simulink model "inverter_w_BESS"  (R2024b)
settings: Solver=VariableStepAuto  StartTime=0.0  StopTime=4  RelTol=1e-3
undefined symbols (not defined in the file): Batt, BatteryCallback, DiscIntNeverNeededParam, gcbh, Q, sps_rtmsupport, Ts, Ts_Control
libraries: simulink x12, spsSeriesRLCBranchLib x7, slpidlib x6, ee_lib x5, nesl_utility x5, eePowerMeasurement x3, powerlib_extras x3, spsCurrentVoltageSimscapeInterfaceLib x3, spsThreePhaseVIMeasurementLib x2, spsCurrentMeasurementLib x2, spsGroundLib x2, spsThreePhaseSeriesRLCBranchLib x2
(part 2 of 2)

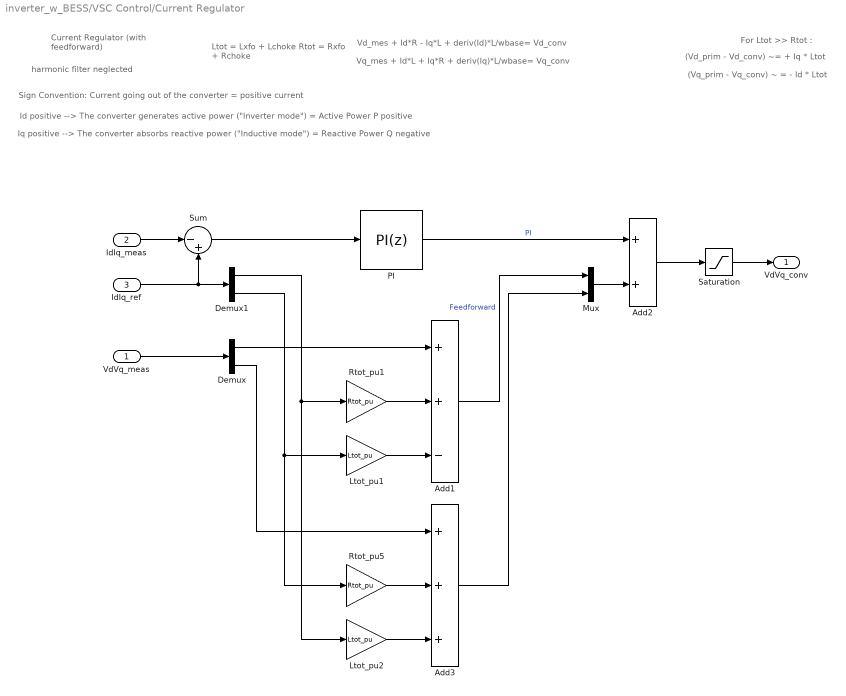
== system inverter_w_BESS/VSC Control/Current Regulator ==
  note: For Ltot >> Rtot :
  note: (Vq_prim - Vq_conv) ~ = - Id * Ltot
  note: (Vd_prim - Vd_conv) ~= + Iq * Ltot
  note: Ltot = Lxfo + Lchoke
      | Rtot = Rxfo + Rchoke
  note: Id positive --> The converter generates active power ("Inverter mode") = Active Power P positive
  note: Iq positive --> The converter absorbs reactive power ("Inductive mode") = Reactive Power Q negative
  note: Sign Convention: Current going out of the converter = positive current
  note: Current Regulator
      | (with feedforward)
  note: Vq_mes + Id*L + Iq*R + deriv(Iq)*L/wbase= Vq_conv
  note: Vd_mes + Id*R - Iq*L + deriv(Id)*L/wbase= Vd_conv
  note: harmonic filter neglected
  VdVq_meas : Inport  PortDimensions=2
  IdIq_meas : Inport  Port=2  PortDimensions=2
  IdIq_ref : Inport  Port=3  PortDimensions=2
  Add1 : Sum  Inputs=++-
  Add2 : Sum
  Add3 : Sum  Inputs=+++
  Demux : Demux  Outputs=2
  Demux1 : Demux  Outputs=2
  Ltot_pu1 : Gain  Gain=Ltot_pu  SaturateOnIntegerOverflow=on  OutDataTypeStr=Inherit: Same as input  ParamDataTypeStr=Inherit: Same as input
  Ltot_pu2 : Gain  Gain=Ltot_pu  SaturateOnIntegerOverflow=on  OutDataTypeStr=Inherit: Same as input  ParamDataTypeStr=Inherit: Same as input
  Mux : Mux  Inputs=2
  PI : slpidlib/PID Controller  Controller=PI  Form=Parallel  TimeDomain=Discrete-time  UseExternalTs=off  SampleTime=Ts  IntegratorMethod=Forward Euler  FilterMethod=Forward Euler  ControllerParametersSource=internal  P=Kp_Ireg  I=Ki_Ireg  UseKiTs=off  D=0  UseExternalDerivativeSource=off  N=100  UseFilter=on  TunerSelectOption=Transfer Function Based (PID Tuner App)  InitialConditionSource=internal  InitialConditionForIntegrator=0  InitialConditionForFilter=0  DifferentiatorICPrevScaledInput=0  ExternalReset=none  TrackingMode=off  Kt=1  LimitOutput=on  SatLimitsSource=internal  UpperSaturationLimit=2  LowerSaturationLimit=-2  LinearizeAsGain=off  AntiWindupMode=none  Kb=1  LimitIntegrator=off  UpperIntegratorSaturationLimit=inf  LowerIntegratorSaturationLimit=-inf  POutMin=[]  POutMax=[]  IOutMin=[]  IOutMax=[]  DOutMin=[]  DOutMax=[]  NOutMin=[]  NOutMax=[]  SumOutMin=[]  SumOutMax=[]  SaturationOutMin=[]  SaturationOutMax=[]  PParamMin=[]  PParamMax=[]  IParamMin=[]  IParamMax=[]  DParamMin=[]  DParamMax=[]  NParamMin=[]  NParamMax=[]  KbParamMin=[]  KbParamMax=[]  KtParamMin=[]  KtParamMax=[]  KbOutMin=[]  KbOutMax=[]  KtOutMin=[]  KtOutMax=[]  IntegratorOutMin=[]  IntegratorOutMax=[]  FilterOutMin=[]  FilterOutMax=[]  SumI1OutMin=[]  SumI1OutMax=[]  SumI2OutMin=[]  SumI2OutMax=[]  SumI3OutMin=[]  SumI3OutMax=[]  SumI4OutMin=[]  SumI4OutMax=[]  SumDOutMin=[]  SumDOutMax=[]  DifferentiatorOutMin=[]  DifferentiatorOutMax=[]  FilterDiffOutCoefMin=[]  FilterDiffOutCoefMax=[]  ReciprocalOutMin=[]  ReciprocalOutMax=[]  SumDenOutMin=[]  SumDenOutMax=[]  SumNumOutMin=[]  SumNumOutMax=[]  DivideOutMin=[]  DivideOutMax=[]  UdiffTsProdOutMin=[]  UdiffTsProdOutMax=[]  NTsProdOutMin=[]  NTsProdOutMax=[]  UintegralTsProdOutMin=[]  UintegralTsProdOutMax=[]  UngainTsProdOutMin=[]  UngainTsProdOutMax=[]  ClampingZeroOutDataTypeStr=Inherit: Inherit via back propagation  ClampingZeroOutMin=[]  ClampingZeroOutMax=[]  FilterDenConstantOutDataTypeStr=Inherit: Inherit via back propagation  FilterDenConstantOutMin=[]  FilterDenConstantOutMax=[]  PCopyOutDataTypeStr=Inherit: Inherit via back propagation  PCopyOutMin=[]  PCopyOutMax=[]  NCopyOutDataTypeStr=Inherit: Inherit via back propagation  NCopyOutMin=[]  NCopyOutMax=[]  IntegratorContinuousStateAttributes=''  IntegratorStateMustResolveToSignalObject=off  IntegratorRTWStateStorageClass=Auto  FilterContinuousStateAttributes=''  FilterStateMustResolveToSignalObject=off  FilterRTWStateStorageClass=Auto  ParallelPVariant=InternalParameters  IdealPVariant=Disabled  IVariant=InternalParameters  DVariant=Disabled  IntegratorVariant=Discrete  SatVariant=Enabled  AWVariant=Passthrough  PCopyVariant=Disabled  TRVariant=Disabled  FdbkBlocksVariant=Forward  IdealPFdbkVariant=Disabled  SatFdbkVariant=Disabled  DerivativeFilterVariant=Disabled  NVariant=Disabled  NCopyVariant=Disabled_SignalSpec  FilterICVariant=Disabled  IntegratorICVariant=InternalICs  ExternalResetVariant=Disabled  TRSumVariant=Passthrough  SumFdbkVariant=Disabled  SumVariant=Sum_PI  TsampFilterVariant=InternalTs  TsampNgainVariant=Passthrough  TsampIntegralVariant=Disabled_SignalSpec  ExternalSaturationOutDataTypeStr=Inherit: Same as second input  DerivativeSourceVariant=Disabled  PreIntVariant=InternalPreInt
  Rtot_pu1 : Gain  Gain=Rtot_pu  SaturateOnIntegerOverflow=on  OutDataTypeStr=Inherit: Same as input  ParamDataTypeStr=Inherit: Same as input
  Rtot_pu5 : Gain  Gain=Rtot_pu  SaturateOnIntegerOverflow=on  OutDataTypeStr=Inherit: Same as input  ParamDataTypeStr=Inherit: Same as input
  Saturation : Saturate  UpperLimit=2  LowerLimit=-2
  Sum : Sum  Inputs=|-+
  VdVq_conv : Outport  VectorParamsAs1DForOutWhenUnconnected=off
  wires:
  Add3/1 -> Mux/2
  Demux/2 -> Add3/1
  Add1/1 -> Mux/1  "Feedforward"
  Ltot_pu2/1 -> Add3/3
  Rtot_pu5/1 -> Add3/2
  Demux1/2 -> Rtot_pu5/1, Ltot_pu1/1
  Ltot_pu1/1 -> Add1/3
  Demux1/1 -> Ltot_pu2/1, Rtot_pu1/1
  Rtot_pu1/1 -> Add1/2
  Demux/1 -> Add1/1
  VdVq_meas/1 -> Demux/1
  Saturation/1 -> VdVq_conv/1
  Add2/1 -> Saturation/1
  IdIq_meas/1 -> Sum/1
  IdIq_ref/1 -> Demux1/1, Sum/2
  Sum/1 -> PI/1
  PI/1 -> Add2/1  "PI"
  Mux/1 -> Add2/2

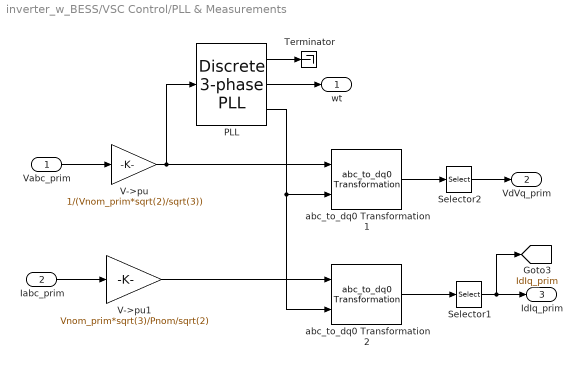
== system inverter_w_BESS/VSC Control/PLL & Measurements ==
  Vabc_prim : Inport
  Iabc_prim : Inport  Port=2
  PLL : powerlib_extras/Discrete  Control Blocks/Discrete 3-phase PLL  Fmin=45  Par_Init="[-0.57  Fnom]"  ParK=[60 1400]  Ts=Ts  AGC=off
  Selector1 : Selector  InputPortWidth=3  IndexOptions=Index vector (dialog)  Indices=[1 2]  OutputSizes=1
  Selector2 : Selector  InputPortWidth=3  IndexOptions=Index vector (dialog)  Indices=[1 2]  OutputSizes=1
  Terminator : Terminator
  V->pu : Gain  Gain=1/(Vnom_prim*sqrt(2)/sqrt(3))  SaturateOnIntegerOverflow=on  OutDataTypeStr=Inherit: Same as input  ParamDataTypeStr=Inherit: Same as input
  V->pu1 : Gain  Gain=Vnom_prim*sqrt(3)/Pnom/sqrt(2)  SaturateOnIntegerOverflow=on  OutDataTypeStr=Inherit: Same as input  ParamDataTypeStr=Inherit: Same as input
  abc_to_dq0 Transformation1 : powerlib_extras/Measurements/abc_to_dq0 Transformation
  abc_to_dq0 Transformation2 : powerlib_extras/Measurements/abc_to_dq0 Transformation
  wt : Outport  VectorParamsAs1DForOutWhenUnconnected=off
  VdVq_prim : Outport  Port=2  VectorParamsAs1DForOutWhenUnconnected=off
  IdIq_prim : Outport  Port=3  VectorParamsAs1DForOutWhenUnconnected=off
  tag scope: IdIq_prim=global
  wires:
  PLL/1 -> Terminator/1
  PLL/3 -> abc_to_dq0 Transformation1/2, abc_to_dq0 Transformation2/2
  Selector1/1 -> IdIq_prim/1, [IdIq_prim]
  Selector2/1 -> VdVq_prim/1
  abc_to_dq0 Transformation1/1 -> Selector2/1
  Iabc_prim/1 -> V->pu1/1
  Vabc_prim/1 -> V->pu/1
  PLL/2 -> wt/1
  abc_to_dq0 Transformation2/1 -> Selector1/1
  V->pu/1 -> abc_to_dq0 Transformation1/1, PLL/1
  V->pu1/1 -> abc_to_dq0 Transformation2/1

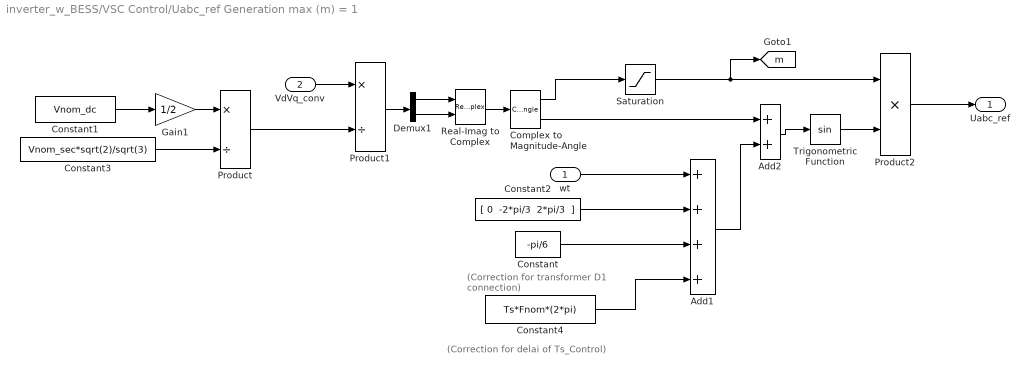
== system inverter_w_BESS/VSC Control/Uabc_ref Generation max (m) = 1 ==
  note: (Correction for delai of Ts_Control)
  note: (Correction for transformer
      |  D1 connection)
  wt : Inport
  VdVq_conv : Inport  Port=2
  Add1 : Sum  Inputs=++++
  Add2 : Sum
  Complex to Magnitude-Angle : ComplexToMagnitudeAngle
  Constant : Constant  Value=-pi/6
  Constant1 : Constant  Value=Vnom_dc
  Constant2 : Constant  Value="[ 0  -2*pi/3  2*pi/3  ]"
  Constant3 : Constant  Value=Vnom_sec*sqrt(2)/sqrt(3)
  Constant4 : Constant  Value=Ts*Fnom*(2*pi)
  Demux1 : Demux  Outputs=2
  Gain1 : Gain  Gain=1/2
  Product : Product  Inputs=*/  RndMeth=Zero
  Product1 : Product  Inputs=*/  RndMeth=Zero
  Product2 : Product  Inputs=**  RndMeth=Zero
  Real-Imag to Complex : RealImagToComplex
  Saturation : Saturate  UpperLimit=1  LowerLimit=0
  Trigonometric Function : Trigonometry
  Uabc_ref : Outport  VectorParamsAs1DForOutWhenUnconnected=off
  tag scope: m=global
  wires:
  Constant4/1 -> Add1/4
  wt/1 -> Add1/1
  Product2/1 -> Uabc_ref/1
  Trigonometric Function/1 -> Product2/2
  Saturation/1 -> Product2/1, [m]
  Add2/1 -> Trigonometric Function/1
  Add1/1 -> Add2/2
  Complex to Magnitude-Angle/2 -> Add2/1
  Product/1 -> Product1/2
  Constant3/1 -> Product/2
  Constant/1 -> Add1/3
  Constant2/1 -> Add1/2
  Demux1/2 -> Real-Imag to Complex/2
  Demux1/1 -> Real-Imag to Complex/1
  Real-Imag to Complex/1 -> Complex to Magnitude-Angle/1
  Gain1/1 -> Product/1
  Product1/1 -> Demux1/1
  VdVq_conv/1 -> Product1/1
  Constant1/1 -> Gain1/1
  Complex to Magnitude-Angle/1 -> Saturation/1

== system inverter_w_BESS/VSC Control/VDC Regulator ==
  Vdc_meas : Inport  PortDimensions=1
  Vdc_ref : Inport  Port=2  PortDimensions=1
  PI : slpidlib/PID Controller  Controller=PI  Form=Parallel  TimeDomain=Discrete-time  UseExternalTs=off  SampleTime=Ts  IntegratorMethod=Trapezoidal  FilterMethod=Forward Euler  ControllerParametersSource=internal  P=Kp_VDCreg  I=Ki_VDCreg  UseKiTs=off  D=0  UseExternalDerivativeSource=off  N=100  UseFilter=on  TunerSelectOption=Transfer Function Based (PID Tuner App)  InitialConditionSource=internal  InitialConditionForIntegrator=0  InitialConditionForFilter=0  DifferentiatorICPrevScaledInput=0  ExternalReset=none  TrackingMode=off  Kt=1  LimitOutput=on  SatLimitsSource=internal  UpperSaturationLimit=1.5  LowerSaturationLimit=-1.5  LinearizeAsGain=off  AntiWindupMode=none  Kb=1  LimitIntegrator=off  UpperIntegratorSaturationLimit=inf  LowerIntegratorSaturationLimit=-inf  POutMin=[]  POutMax=[]  IOutMin=[]  IOutMax=[]  DOutMin=[]  DOutMax=[]  NOutMin=[]  NOutMax=[]  SumOutMin=[]  SumOutMax=[]  SaturationOutMin=[]  SaturationOutMax=[]  PParamMin=[]  PParamMax=[]  IParamMin=[]  IParamMax=[]  DParamMin=[]  DParamMax=[]  NParamMin=[]  NParamMax=[]  KbParamMin=[]  KbParamMax=[]  KtParamMin=[]  KtParamMax=[]  KbOutMin=[]  KbOutMax=[]  KtOutMin=[]  KtOutMax=[]  IntegratorOutMin=[]  IntegratorOutMax=[]  FilterOutMin=[]  FilterOutMax=[]  SumI1OutMin=[]  SumI1OutMax=[]  SumI2OutMin=[]  SumI2OutMax=[]  SumI3OutMin=[]  SumI3OutMax=[]  SumI4OutMin=[]  SumI4OutMax=[]  SumDOutMin=[]  SumDOutMax=[]  DifferentiatorOutMin=[]  DifferentiatorOutMax=[]  FilterDiffOutCoefMin=[]  FilterDiffOutCoefMax=[]  ReciprocalOutMin=[]  ReciprocalOutMax=[]  SumDenOutMin=[]  SumDenOutMax=[]  SumNumOutMin=[]  SumNumOutMax=[]  DivideOutMin=[]  DivideOutMax=[]  UdiffTsProdOutMin=[]  UdiffTsProdOutMax=[]  NTsProdOutMin=[]  NTsProdOutMax=[]  UintegralTsProdOutMin=[]  UintegralTsProdOutMax=[]  UngainTsProdOutMin=[]  UngainTsProdOutMax=[]  ClampingZeroOutDataTypeStr=Inherit: Inherit via back propagation  ClampingZeroOutMin=[]  ClampingZeroOutMax=[]  FilterDenConstantOutDataTypeStr=Inherit: Inherit via back propagation  FilterDenConstantOutMin=[]  FilterDenConstantOutMax=[]  PCopyOutDataTypeStr=Inherit: Inherit via back propagation  PCopyOutMin=[]  PCopyOutMax=[]  NCopyOutDataTypeStr=Inherit: Inherit via back propagation  NCopyOutMin=[]  NCopyOutMax=[]  IntegratorContinuousStateAttributes=''  IntegratorStateMustResolveToSignalObject=off  IntegratorRTWStateStorageClass=Auto  FilterContinuousStateAttributes=''  FilterStateMustResolveToSignalObject=off  FilterRTWStateStorageClass=Auto  ParallelPVariant=InternalParameters  IdealPVariant=Disabled  IVariant=InternalParameters  DVariant=Disabled  IntegratorVariant=Discrete  SatVariant=Enabled  AWVariant=Passthrough  PCopyVariant=Disabled  TRVariant=Disabled  FdbkBlocksVariant=Forward  IdealPFdbkVariant=Disabled  SatFdbkVariant=Disabled  DerivativeFilterVariant=Disabled  NVariant=Disabled  NCopyVariant=Disabled_SignalSpec  FilterICVariant=Disabled  IntegratorICVariant=InternalICs  ExternalResetVariant=Disabled  TRSumVariant=Passthrough  SumFdbkVariant=Disabled  SumVariant=Sum_PI  TsampFilterVariant=InternalTs  TsampNgainVariant=Passthrough  TsampIntegralVariant=Disabled_SignalSpec  ExternalSaturationOutDataTypeStr=Inherit: Same as second input  DerivativeSourceVariant=Disabled  PreIntVariant=InternalPreInt
  Rtot_pu3 : Gain  Gain=1/Vnom_dc  SaturateOnIntegerOverflow=on  OutDataTypeStr=Inherit: Same as input  ParamDataTypeStr=Inherit: Same as input
  Sum : Sum  Inputs=|+-
  Id_ref : Outport  SampleTime=Ts  InitialOutput=0  VectorParamsAs1DForOutWhenUnconnected=off
  tag scope: Id_ref=global, Vdc_ref=global
  wires:
  Rtot_pu3/1 -> PI/1
  Vdc_ref/1 -> [Vdc_ref], Sum/2
  Vdc_meas/1 -> Sum/1
  Sum/1 -> Rtot_pu3/1
  PI/1 -> [Id_ref], Id_ref/1

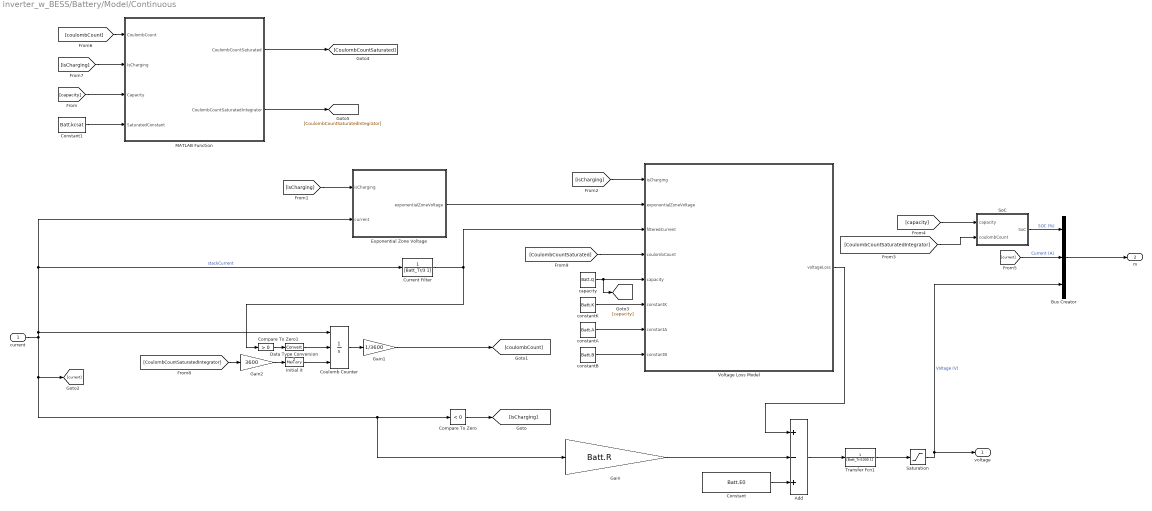
== system inverter_w_BESS/Battery/Model/Continuous ==
  current : Inport
  Add : Sum  Inputs=+-+
  Bus Creator : BusCreator  Inputs=3
  Compare To Zero : simulink/Logic and Bit Operations/Compare To Zero  relop=<  OutDataTypeStr=boolean
  Compare To Zero1 : simulink/Logic and Bit Operations/Compare To Zero  relop=>  OutDataTypeStr=uint8
  Constant : Constant  Value=Batt.E0
  Constant1 : Constant  Value=Batt.kcsat
  Coulomb Counter : Integrator  ExternalReset=rising  InitialConditionSource=external  InitialCondition=(1-SOC/100)*Q*3600  LimitOutput=on  UpperSaturationLimit=Batt.Q*3600
  Current Filter : TransferFcn  Denominator=[Batt_Tr/3 1]
  Data Type Conversion2 : DataTypeConversion  SaturateOnIntegerOverflow=off  RndMeth=Floor
  Exponential Zone Voltage : Subsystem
  Gain : Gain  Gain=Batt.R
  Gain1 : Gain  Gain=1/3600
  Gain2 : Gain  Gain=3600
  Initial it : Memory  InitialCondition=(1-SOC/100)*Batt.Q*(1/Batt.lambda)*3600
  MATLAB Function : MATLAB Function  TreatAsAtomicUnit=on
  Saturation : Saturate  UpperLimit=2*Batt.E0  LowerLimit=0
  SoC : Subsystem
  Transfer Fcn1 : TransferFcn  Denominator=[Batt_Tr/1000 1]
  Voltage Loss Model : Subsystem  Variant=on  VariantControlMode=label  LabelModeActiveChoice=lead_acid
  capacity : Constant  Value=Batt.Q
  constantA : Constant  Value=Batt.A
  constantB : Constant  Value=Batt.B
  constantK : Constant  Value=Batt.K
  voltage : Outport
  m : Outport  Port=2
  wires:
  [isCharging] -> MATLAB Function/2(IsCharging)
  [coulombCount] -> MATLAB Function/1(CoulombCount)
  Constant1/1 -> MATLAB Function/4(SaturatedConstant)
  [capacity] -> MATLAB Function/3(Capacity)
  MATLAB Function/2(CoulombCountSaturatedIntegrator) -> [CoulombCountSaturatedIntegrator]
  MATLAB Function/1(CoulombCountSaturated) -> [CoulombCountSaturated]
  [CoulombCountSaturated] -> Voltage Loss Model/4(coulombCount)
  Current Filter/1 -> Voltage Loss Model/3(filteredCurrent), Compare To Zero1/1
  Initial it/1 -> Coulomb Counter/3
  Compare To Zero1/1 -> Data Type Conversion2/1
  Data Type Conversion2/1 -> Coulomb Counter/2
  Gain2/1 -> Initial it/1
  Coulomb Counter/1 -> Gain1/1
  [CoulombCountSaturatedIntegrator] -> Gain2/1
  Compare To Zero/1 -> [isCharging]
  Transfer Fcn1/1 -> Saturation/1
  Gain1/1 -> [coulombCount]
  constantK/1 -> Voltage Loss Model/6(constantK)
  Bus Creator/1 -> m/1
  [isCharging] -> Exponential Zone Voltage/1(isCharging)
  Saturation/1 -> Bus Creator/3, voltage/1  "Voltage (V)"
  [isCharging] -> Voltage Loss Model/1(isCharging)
  SoC/1(SoC) -> Bus Creator/1  "SOC (%)"
  current/1 -> [current], Gain/1, Compare To Zero/1, Exponential Zone Voltage/2(current), Current Filter/1, Coulomb Counter/1  "stackCurrent"
  capacity/1 -> [capacity], Voltage Loss Model/5(capacity)
  constantA/1 -> Voltage Loss Model/7(constantA)
  [CoulombCountSaturatedIntegrator] -> SoC/2(coulombCount)
  Exponential Zone Voltage/1(exponentialZoneVoltage) -> Voltage Loss Model/2(exponentialZoneVoltage)
  [capacity] -> SoC/1(capacity)
  [current] -> Bus Creator/2  "Current (A)"
  Constant/1 -> Add/3
  constantB/1 -> Voltage Loss Model/8(constantB)
  Gain/1 -> Add/2
  Voltage Loss Model/1(voltageLoss) -> Add/1
  Add/1 -> Transfer Fcn1/1

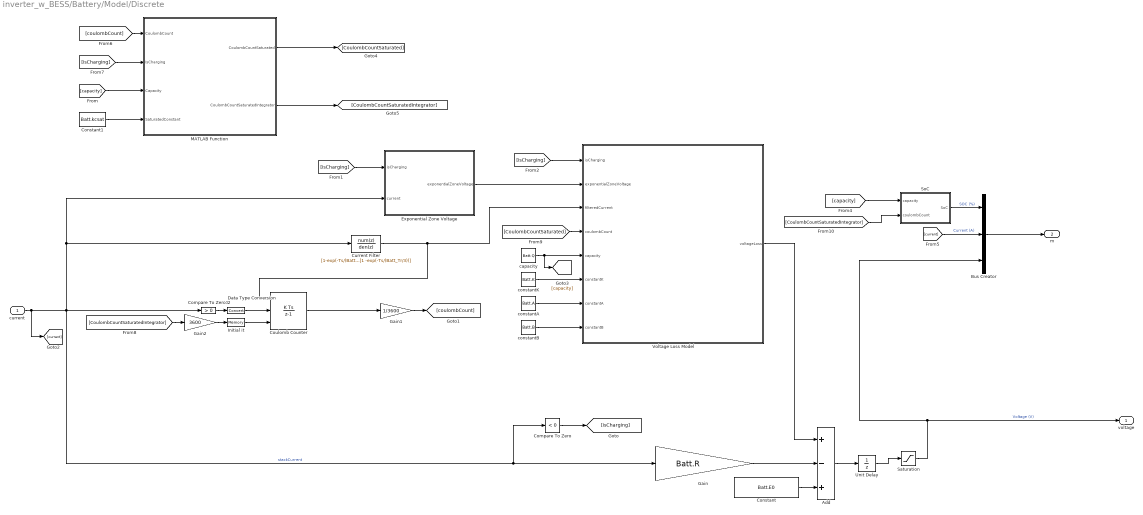
== system inverter_w_BESS/Battery/Model/Discrete ==
  current : Inport
  Add : Sum  Inputs=+-+
  Bus Creator : BusCreator  Inputs=3
  Compare To Zero : simulink/Logic and Bit Operations/Compare To Zero  relop=<  OutDataTypeStr=boolean
  Compare To Zero1 : simulink/Logic and Bit Operations/Compare To Zero  relop=>  OutDataTypeStr=uint8
  Constant : Constant  Value=Batt.E0
  Constant1 : Constant  Value=Batt.kcsat
  Coulomb Counter : DiscreteIntegrator  ExternalReset=rising  InitialConditionSource=external  SampleTime=-1  LimitOutput=on  UpperSaturationLimit=Batt.Q*3600  ICPrevOutput=DiscIntNeverNeededParam  ICPrevScaledInput=DiscIntNeverNeededParam
  Current Filter : DiscreteTransferFcn  Numerator=[1-exp(-Ts/(Batt_Tr/3))]  Denominator=[1 -exp(-Ts/(Batt_Tr/3))]
  Data Type Conversion2 : DataTypeConversion  SaturateOnIntegerOverflow=off  RndMeth=Floor
  Exponential Zone Voltage : Subsystem
  Gain : Gain  Gain=Batt.R
  Gain1 : Gain  Gain=1/3600
  Gain2 : Gain  Gain=3600
  Initial it : Memory  InitialCondition=(1-SOC/100)*Batt.Q*(1/Batt.lambda)*3600
  MATLAB Function : MATLAB Function  TreatAsAtomicUnit=on
  Saturation : Saturate  UpperLimit=2*Batt.E0  LowerLimit=0
  SoC : Subsystem
  Unit Delay : UnitDelay  SampleTime=-1  HasFrameUpgradeWarning=on
  Voltage Loss Model : Subsystem  Variant=on  VariantControlMode=label  LabelModeActiveChoice=lithium_ion
  capacity : Constant  Value=Batt.Q
  constantA : Constant  Value=Batt.A
  constantB : Constant  Value=Batt.B
  constantK : Constant  Value=Batt.K
  voltage : Outport
  m : Outport  Port=2
  wires:
  [capacity] -> MATLAB Function/3(Capacity)
  Constant1/1 -> MATLAB Function/4(SaturatedConstant)
  MATLAB Function/2(CoulombCountSaturatedIntegrator) -> [CoulombCountSaturatedIntegrator]
  [isCharging] -> MATLAB Function/2(IsCharging)
  MATLAB Function/1(CoulombCountSaturated) -> [CoulombCountSaturated]
  [coulombCount] -> MATLAB Function/1(CoulombCount)
  [CoulombCountSaturated] -> Voltage Loss Model/4(coulombCount)
  [CoulombCountSaturatedIntegrator] -> Gain2/1
  Coulomb Counter/1 -> Gain1/1
  Initial it/1 -> Coulomb Counter/3
  Compare To Zero1/1 -> Data Type Conversion2/1
  Gain2/1 -> Initial it/1
  Data Type Conversion2/1 -> Coulomb Counter/2
  Current Filter/1 -> Voltage Loss Model/3(filteredCurrent), Coulomb Counter/1
  Unit Delay/1 -> Saturation/1
  Add/1 -> Unit Delay/1
  Voltage Loss Model/1(voltageLoss) -> Add/1
  Gain/1 -> Add/2
  constantB/1 -> Voltage Loss Model/8(constantB)
  Constant/1 -> Add/3
  [current] -> Bus Creator/2  "Current (A)"
  [capacity] -> SoC/1(capacity)
  Exponential Zone Voltage/1(exponentialZoneVoltage) -> Voltage Loss Model/2(exponentialZoneVoltage)
  [CoulombCountSaturatedIntegrator] -> SoC/2(coulombCount)
  Compare To Zero/1 -> [isCharging]
  constantA/1 -> Voltage Loss Model/7(constantA)
  capacity/1 -> Voltage Loss Model/5(capacity), [capacity]
  current/1 -> Exponential Zone Voltage/2(current), Current Filter/1, Compare To Zero1/1, Gain/1, Compare To Zero/1, [current]  "stackCurrent"
  SoC/1(SoC) -> Bus Creator/1  "SOC (%)"
  [isCharging] -> Voltage Loss Model/1(isCharging)
  Saturation/1 -> voltage/1, Bus Creator/3  "Voltage (V)"
  [isCharging] -> Exponential Zone Voltage/1(isCharging)
  Bus Creator/1 -> m/1
  constantK/1 -> Voltage Loss Model/6(constantK)
  Gain1/1 -> [coulombCount]

== system inverter_w_BESS/Battery/Model/Continuous/Exponential Zone Voltage ==
  isCharging : Inport
  current : Inport  Port=2
  Abs : Abs  SaturateOnIntegerOverflow=off
  Add1 : Sum  Inputs=-+
  Cast To Double : DataTypeConversion  OutDataTypeStr=double  SaturateOnIntegerOverflow=off  RndMeth=Floor
  Gain : Gain  Gain=Batt.B/3600
  Gain1 : Gain  Gain=Batt.A
  Integrator2 : Integrator  InitialCondition=Batt.A*exp(-Batt.B*(1-SOC/100)*Batt.Q)
  Product : Product
  Product1 : Product
  exponentialZoneVoltage : Outport
  wires:
  Cast To Double/1 -> Gain1/1
  isCharging/1 -> Cast To Double/1
  Gain1/1 -> Product/2
  Product/1 -> Add1/2
  Integrator2/1 -> exponentialZoneVoltage/1, Product1/1
  Product1/1 -> Add1/1
  Gain/1 -> Product1/2, Product/1
  current/1 -> Abs/1
  Add1/1 -> Integrator2/1
  Abs/1 -> Gain/1

== system inverter_w_BESS/Battery/Model/Continuous/SoC ==
  capacity : Inport
  coulombCount : Inport  Port=2
  Fcn : Fcn  Expr=(u(1)-u(2))/u(1)
  Gain1 : Gain  Gain=100
  Mux : Mux  Inputs=2
  Saturation : Saturate  UpperLimit=100  LowerLimit=0
  SoC : Outport
  wires:
  Fcn/1 -> Gain1/1
  Gain1/1 -> Saturation/1
  Saturation/1 -> SoC/1
  Mux/1 -> Fcn/1
  capacity/1 -> Mux/1
  coulombCount/1 -> Mux/2

== system inverter_w_BESS/Battery/Model/Continuous/Voltage Loss Model ==
  isCharging : Inport
  exponentialZoneVoltage : Inport  Port=2
  filteredCurrent : Inport  Port=3
  coulombCount : Inport  Port=4
  capacity : Inport  Port=5
  constantK : Inport  Port=6
  constantA : Inport  Port=7
  constantB : Inport  Port=8
  Lead Acid : Subsystem  VariantControl=lead_acid
  Lithium Ion : Subsystem  VariantControl=lithium_ion
  Nickel : Subsystem  VariantControl=nickel
  voltageLoss : Outport

== system inverter_w_BESS/Battery/Model/Discrete/Exponential Zone Voltage ==
  isCharging : Inport
  current : Inport  Port=2
  Abs : Abs  SaturateOnIntegerOverflow=off
  Add1 : Sum  Inputs=-+
  Cast To Double : DataTypeConversion  OutDataTypeStr=double  SaturateOnIntegerOverflow=off  RndMeth=Floor
  Discrete-Time Integrator : DiscreteIntegrator  InitialCondition=Batt.A*exp(-Batt.B*(1-SOC/100)*Batt.Q)  SampleTime=-1  ICPrevOutput=DiscIntNeverNeededParam  ICPrevScaledInput=DiscIntNeverNeededParam
  Gain : Gain  Gain=Batt.B/3600
  Gain1 : Gain  Gain=Batt.A
  Product : Product
  Product1 : Product
  exponentialZoneVoltage : Outport
  wires:
  Cast To Double/1 -> Gain1/1
  Abs/1 -> Gain/1
  Add1/1 -> Discrete-Time Integrator/1
  current/1 -> Abs/1
  Gain/1 -> Product/1, Product1/2
  Product1/1 -> Add1/1
  Discrete-Time Integrator/1 -> Product1/1, exponentialZoneVoltage/1
  Product/1 -> Add1/2
  isCharging/1 -> Cast To Double/1
  Gain1/1 -> Product/2

== system inverter_w_BESS/Battery/Model/Discrete/SoC ==
  capacity : Inport
  coulombCount : Inport  Port=2
  Fcn : Fcn  Expr=(u(1)-u(2))/u(1)
  Gain1 : Gain  Gain=100
  Mux : Mux  Inputs=2
  Saturation : Saturate  UpperLimit=100  LowerLimit=0
  SoC : Outport
  wires:
  coulombCount/1 -> Mux/2
  capacity/1 -> Mux/1
  Mux/1 -> Fcn/1
  Saturation/1 -> SoC/1
  Gain1/1 -> Saturation/1
  Fcn/1 -> Gain1/1

== system inverter_w_BESS/Battery/Model/Discrete/Voltage Loss Model ==
  isCharging : Inport
  exponentialZoneVoltage : Inport  Port=2
  filteredCurrent : Inport  Port=3
  coulombCount : Inport  Port=4
  capacity : Inport  Port=5
  constantK : Inport  Port=6
  constantA : Inport  Port=7
  constantB : Inport  Port=8
  Lead Acid : Subsystem  VariantControl=lead_acid
  Lithium Ion : Subsystem  VariantControl=lithium_ion
  Nickel : Subsystem  VariantControl=nickel
  voltageLoss : Outport

== system inverter_w_BESS/Battery/Model/Continuous/Voltage Loss Model/Lead Acid ==
  isCharging : Inport
  exponentialZoneVoltage : Inport  Port=2
  filteredCurrent : Inport  Port=3
  coulombCount : Inport  Port=4
  capacity : Inport  Port=5
  constantK : Inport  Port=6
  MATLAB Function12 : MATLAB Function  TreatAsAtomicUnit=on
  voltageLoss : Outport
  wires:
  MATLAB Function12/1(VoltageLoss) -> voltageLoss/1
  isCharging/1 -> MATLAB Function12/1(IsCharging)
  exponentialZoneVoltage/1 -> MATLAB Function12/2(ExponentialZoneVoltage)
  filteredCurrent/1 -> MATLAB Function12/3(FilteredCurrent)
  coulombCount/1 -> MATLAB Function12/4(CoulombCount)
  capacity/1 -> MATLAB Function12/5(Capacity)
  constantK/1 -> MATLAB Function12/6(ConstantK)

== system inverter_w_BESS/Battery/Model/Continuous/Voltage Loss Model/Lithium Ion ==
  isCharging : Inport
  exponentialZoneVoltage : Inport  Port=2
  filteredCurrent : Inport  Port=3
  coulombCount : Inport  Port=4
  capacity : Inport  Port=5
  constantK : Inport  Port=6
  constantA : Inport  Port=7
  constantB : Inport  Port=8
  MATLAB Function : MATLAB Function  TreatAsAtomicUnit=on
  voltageLoss : Outport
  wires:
  capacity/1 -> MATLAB Function/5(Capacity)
  MATLAB Function/1(VoltageLoss) -> voltageLoss/1
  constantK/1 -> MATLAB Function/6(ConstantK)
  exponentialZoneVoltage/1 -> MATLAB Function/2(ExponentialZoneVoltage)
  constantA/1 -> MATLAB Function/7(ConstantA)
  filteredCurrent/1 -> MATLAB Function/3(FilteredCurrent)
  constantB/1 -> MATLAB Function/8(ConstantB)
  coulombCount/1 -> MATLAB Function/4(CoulombCount)
  isCharging/1 -> MATLAB Function/1(IsCharging)

== system inverter_w_BESS/Battery/Model/Continuous/Voltage Loss Model/Nickel ==
  isCharging : Inport
  exponentialZoneVoltage : Inport  Port=2
  filteredCurrent : Inport  Port=3
  coulombCount : Inport  Port=4
  capacity : Inport  Port=5
  constantK : Inport  Port=6
  MATLAB Function : MATLAB Function  TreatAsAtomicUnit=on
  voltageLoss : Outport
  wires:
  capacity/1 -> MATLAB Function/5(Capacity)
  constantK/1 -> MATLAB Function/6(ConstantK)
  MATLAB Function/1(VoltageLoss) -> voltageLoss/1
  isCharging/1 -> MATLAB Function/1(IsCharging)
  exponentialZoneVoltage/1 -> MATLAB Function/2(ExponentialZoneVoltage)
  filteredCurrent/1 -> MATLAB Function/3(FilteredCurrent)
  coulombCount/1 -> MATLAB Function/4(CoulombCount)

== system inverter_w_BESS/Battery/Model/Discrete/Voltage Loss Model/Lead Acid ==
  isCharging : Inport
  exponentialZoneVoltage : Inport  Port=2
  filteredCurrent : Inport  Port=3
  coulombCount : Inport  Port=4
  capacity : Inport  Port=5
  constantK : Inport  Port=6
  MATLAB Function12 : MATLAB Function  TreatAsAtomicUnit=on
  voltageLoss : Outport
  wires:
  constantK/1 -> MATLAB Function12/6(ConstantK)
  capacity/1 -> MATLAB Function12/5(Capacity)
  coulombCount/1 -> MATLAB Function12/4(CoulombCount)
  filteredCurrent/1 -> MATLAB Function12/3(FilteredCurrent)
  exponentialZoneVoltage/1 -> MATLAB Function12/2(ExponentialZoneVoltage)
  MATLAB Function12/1(VoltageLoss) -> voltageLoss/1
  isCharging/1 -> MATLAB Function12/1(IsCharging)

== system inverter_w_BESS/Battery/Model/Discrete/Voltage Loss Model/Lithium Ion ==
  isCharging : Inport
  exponentialZoneVoltage : Inport  Port=2
  filteredCurrent : Inport  Port=3
  coulombCount : Inport  Port=4
  capacity : Inport  Port=5
  constantK : Inport  Port=6
  constantA : Inport  Port=7
  constantB : Inport  Port=8
  MATLAB Function : MATLAB Function  TreatAsAtomicUnit=on
  voltageLoss : Outport
  wires:
  isCharging/1 -> MATLAB Function/1(IsCharging)
  coulombCount/1 -> MATLAB Function/4(CoulombCount)
  constantB/1 -> MATLAB Function/8(ConstantB)
  filteredCurrent/1 -> MATLAB Function/3(FilteredCurrent)
  constantA/1 -> MATLAB Function/7(ConstantA)
  exponentialZoneVoltage/1 -> MATLAB Function/2(ExponentialZoneVoltage)
  constantK/1 -> MATLAB Function/6(ConstantK)
  MATLAB Function/1(VoltageLoss) -> voltageLoss/1
  capacity/1 -> MATLAB Function/5(Capacity)

== system inverter_w_BESS/Battery/Model/Discrete/Voltage Loss Model/Nickel ==
  isCharging : Inport
  exponentialZoneVoltage : Inport  Port=2
  filteredCurrent : Inport  Port=3
  coulombCount : Inport  Port=4
  capacity : Inport  Port=5
  constantK : Inport  Port=6
  MATLAB Function : MATLAB Function  TreatAsAtomicUnit=on
  voltageLoss : Outport
  wires:
  coulombCount/1 -> MATLAB Function/4(CoulombCount)
  filteredCurrent/1 -> MATLAB Function/3(FilteredCurrent)
  exponentialZoneVoltage/1 -> MATLAB Function/2(ExponentialZoneVoltage)
  isCharging/1 -> MATLAB Function/1(IsCharging)
  MATLAB Function/1(VoltageLoss) -> voltageLoss/1
  constantK/1 -> MATLAB Function/6(ConstantK)
  capacity/1 -> MATLAB Function/5(Capacity)

== matlab function inverter_w_BESS/Battery/Model/Discrete/Voltage Loss Model/Nickel/MATLAB Function ==
  data: IsCharging input; VoltageLoss output; ExponentialZoneVoltage input; FilteredCurrent input; CoulombCount input; Capacity input; ConstantK input
function VoltageLoss = calculateVoltageLossNickel(IsCharging,ExponentialZoneVoltage,FilteredCurrent,CoulombCount,Capacity,ConstantK)

VoltageLoss = calculateVoltageLossNickel(IsCharging,ExponentialZoneVoltage,FilteredCurrent,CoulombCount,Capacity,ConstantK);

end

== matlab function inverter_w_BESS/BATT chg-dshg logic/MATLAB Function1 ==
  data: Vdc input; Vbatt input; I_batt_meas input; I_batt_ref_mag input; D output; mode input
% MATLAB implementation of unified PI control for bidirectional DC-DC converter
% Modified to allow manual toggle between charging (mode = 0) and discharging (mode = 1)

function D = bidirectional_controller(Vdc, Vbatt, I_batt_meas, I_batt_ref_mag, mode)
%#codegen

% Limits
Imax_charge = 50;
Imax_discharge = -50;

% PI gains
Kp = 0.01;
Ki = 0.05;
persistent integral_error
if isempty(integral_error)
    integral_error = 0;
end

% Adjust reference sign based on mode
if mode == 0
    I_batt_ref = I_batt_ref_mag;      % Charging
elseif mode == 1
    I_batt_ref = -I_batt_ref_mag;     % Discharging
else
    I_batt_ref = 0;
end

% Clamp current reference
I_batt_ref = max(min(I_batt_ref, Imax_charge), Imax_discharge);

% PI control
error = I_batt_ref - I_batt_meas;
dt = 1e-4;
integral_error = integral_error + error * dt;
PI_output = Kp * error + Ki * integral_error;

% Base duty calculation
if mode == 0
    D_base = Vbatt / Vdc;             % Buck mode
elseif mode == 1
    D_base = 1 - Vbatt / Vdc;         % Boost mode
else
    D_base = 0;
end

% Total duty
D = D_base + PI_output;
D = min(max(D, 0.05), 0.95);

end

== matlab function inverter_w_BESS/Battery/Model/Continuous/Voltage Loss Model/Lead Acid/MATLAB Function12 ==
  data: IsCharging input; VoltageLoss output; ExponentialZoneVoltage input; FilteredCurrent input; CoulombCount input; Capacity input; ConstantK input
function VoltageLoss = calculateVoltageLossLeadAcid(IsCharging,ExponentialZoneVoltage,FilteredCurrent,CoulombCount,Capacity,ConstantK)

% Copyright 2024 The MathWorks, Inc. 
VoltageLoss = calculateVoltageLossLeadAcid(IsCharging,ExponentialZoneVoltage,FilteredCurrent,CoulombCount,Capacity,ConstantK);

end

== matlab function inverter_w_BESS/MPPT/MATLAB Function1 ==
  data: ipv input; Vmpp output; vpv input
function Vmpp = mppt_inccond(ipv, vpv)
    % Incremental Conductance MPPT to output Vmpp
    % Inputs:
    %   ipv - PV current (A)
    %   vpv - PV voltage (V)
    % Output:
    %   Vmpp - Maximum power point voltage (V)

    % Persistent variables to store previous states
    persistent I_prev V_prev Vpv_ref_prev

    % Initialize persistent variables
    if isempty(I_prev)
        I_prev = ipv;
        V_prev = vpv;
        Vpv_ref_prev = 364.5;     % Initial guess near Vmpp
    end

    % Parameters
    delta_Vpv = 1;           % Step size for Vpv_ref adjustment
    tol = 1e-4;                % MPP detection tolerance
    v_min = 5;                 % Minimum voltage threshold

    % Handle invalid inputs
    if isnan(ipv) || isnan(vpv) || vpv < v_min
        Vmpp = Vpv_ref_prev;
        return;
    end

    % Incremental Conductance Algorithm
    delta_I = ipv - I_prev;
    delta_V = vpv - V_prev;

    if abs(delta_V) < 1e-4
        if delta_I > 1e-3
            Vpv_ref = Vpv_ref_prev + delta_Vpv;
        elseif delta_I < -1e-3
            Vpv_ref = Vpv_ref_prev - delta_Vpv;
        else
            Vpv_ref = Vpv_ref_prev;
        end
    else
        inst_cond = ipv / vpv;
        inc_cond = delta_I / delta_V;

        if abs(inc_cond + inst_cond) < tol
            Vpv_ref = Vpv_ref_prev;
        elseif inc_cond > -inst_cond
            Vpv_ref = Vpv_ref_prev + delta_Vpv;
        else
            Vpv_ref = Vpv_ref_prev - delta_Vpv;
        end
    end

    % Clamp Vpv_ref to safe range
    Vpv_ref = min(426.5, max(150, Vpv_ref));

    % Output Vmpp
    Vmpp = Vpv_ref;

    % Update states
    I_prev = ipv;
    V_prev = vpv;
    Vpv_ref_prev = Vpv_ref;
end

== matlab function inverter_w_BESS/MPPT/MATLAB Function2 ==
  data: ipv input; D output; vpv input
function D = inccond_mppt(ipv, vpv)
    % Incremental Conductance MPPT algorithm for PV system (optimized for boost converter)
    % Inputs: ipv - PV current (A), vpv - PV voltage (V)
    % Output: D - Duty cycle (0.2 to 0.392)

    persistent I_prev V_prev D_prev;
    if isempty(I_prev)
        I_prev = 0;
        V_prev = 0; % Initial PV voltage (based on Vmp = 364.5 V)
        D_prev = 0; % Initial duty cycle
    end

    delta_D = 0.008; % Step size for duty cycle adjustment
    D_min = 0.391;     % Minimum duty cycle
    D_max = 0.48;     % Maximum duty cycle
    tol = 1e-3;      % Tolerance for MPP detection
    v_min = 1e-3;    % Minimum voltage threshold

    % Check for invalid inputs
    if isnan(ipv) || isnan(vpv) || ipv < 0 || vpv < v_min
        D = D_prev;
        return;
    end

    % Calculate incremental changes
    delta_I = ipv - I_prev;
    delta_V = vpv - V_prev;

    % Handle small delta_V
    if abs(delta_V) < 1e-4
        if delta_I > 1e-4
            D = D_prev - delta_D; % Increase voltage (decrease D for boost)
        elseif delta_I < -1e-4
            D = D_prev + delta_D; % Decrease voltage (increase D for boost)
        else
            D = D_prev; % No change
        end
    else
        % Calculate instantaneous and incremental conductance
        inst_cond = ipv / vpv; % I/V
        inc_cond = delta_I / delta_V; % dI/dV

        % Compare incremental and instantaneous conductance
        if abs(inc_cond + inst_cond) < tol
            D = D_prev; % At MPP
        elseif inc_cond > -inst_cond
            D = D_prev - delta_D; % Left of MPP, increase voltage (decrease D for boost)
        else
            D = D_prev + delta_D; % Right of MPP, decrease voltage (increase D for boost)
        end
    end

    % Limit duty cycle
    D = min(D_max, max(D_min, D));

    % Update previous values
    I_prev = ipv;
    V_prev = vpv;
    D_prev = D;
end

== matlab function inverter_w_BESS/Battery/Model/Continuous/Voltage Loss Model/Lithium Ion/MATLAB Function ==
  data: IsCharging input; VoltageLoss output; ExponentialZoneVoltage input; FilteredCurrent input; CoulombCount input; Capacity input; ConstantK input; ConstantA input; ConstantB input
function VoltageLoss = calculateVoltageLossLithiumIon(IsCharging,ExponentialZoneVoltage,FilteredCurrent,CoulombCount,Capacity,ConstantK,ConstantA,ConstantB)

    VoltageLoss = calculateVoltageLossLithiumIon(IsCharging,ExponentialZoneVoltage,FilteredCurrent,CoulombCount,Capacity,ConstantK,ConstantA,ConstantB);

end

== matlab function inverter_w_BESS/Battery/Model/Continuous/Voltage Loss Model/Nickel/MATLAB Function ==
  data: IsCharging input; VoltageLoss output; ExponentialZoneVoltage input; FilteredCurrent input; CoulombCount input; Capacity input; ConstantK input
function VoltageLoss = calculateVoltageLossNickel(IsCharging,ExponentialZoneVoltage,FilteredCurrent,CoulombCount,Capacity,ConstantK)

VoltageLoss = calculateVoltageLossNickel(IsCharging,ExponentialZoneVoltage,FilteredCurrent,CoulombCount,Capacity,ConstantK);
%VoltageLoss = BatteryCalculateVoltageLoss('Nickel',IsCharging,ExponentialZoneVoltage,FilteredCurrent,CoulombCount,Capacity,ConstantK);

end

== matlab function inverter_w_BESS/Battery/Model/Discrete/Voltage Loss Model/Lead Acid/MATLAB Function12 ==
  data: IsCharging input; VoltageLoss output; ExponentialZoneVoltage input; FilteredCurrent input; CoulombCount input; Capacity input; ConstantK input
function VoltageLoss = calculateVoltageLossLeadAcid(IsCharging,ExponentialZoneVoltage,FilteredCurrent,CoulombCount,Capacity,ConstantK)

% Copyright 2024 The MathWorks, Inc.

VoltageLoss = calculateVoltageLossLeadAcid(IsCharging,ExponentialZoneVoltage,FilteredCurrent,CoulombCount,Capacity,ConstantK);

end

== matlab function inverter_w_BESS/Battery/Model/Continuous/MATLAB Function ==
  data: CoulombCount input; CoulombCountSaturated output; IsCharging input; Capacity input; SaturatedConstant input; CoulombCountSaturatedIntegrator output
function [CoulombCountSaturated,CoulombCountSaturatedIntegrator] = calculateCoulombSaturation(CoulombCount,IsCharging,Capacity,SaturatedConstant)

    [CoulombCountSaturated,CoulombCountSaturatedIntegrator] = calculateCoulombSaturation(CoulombCount,IsCharging,Capacity,SaturatedConstant);

end

== matlab function inverter_w_BESS/Battery/Model/Discrete/MATLAB Function ==
  data: CoulombCount input; CoulombCountSaturated output; IsCharging input; Capacity input; SaturatedConstant input; CoulombCountSaturatedIntegrator output
function [CoulombCountSaturated,CoulombCountSaturatedIntegrator] = calculateCoulombSaturation(CoulombCount,IsCharging,Capacity,SaturatedConstant)

    [CoulombCountSaturated,CoulombCountSaturatedIntegrator] = calculateCoulombSaturation(CoulombCount,IsCharging,Capacity,SaturatedConstant);

end

== matlab function inverter_w_BESS/Battery/Model/Discrete/Voltage Loss Model/Lithium Ion/MATLAB Function ==
  data: IsCharging input; VoltageLoss output; ExponentialZoneVoltage input; FilteredCurrent input; CoulombCount input; Capacity input; ConstantK input; ConstantA input; ConstantB input
function VoltageLoss = calculateVoltageLossLithiumIon(IsCharging,ExponentialZoneVoltage,FilteredCurrent,CoulombCount,Capacity,ConstantK,ConstantA,ConstantB)

    VoltageLoss = calculateVoltageLossLithiumIon(IsCharging,ExponentialZoneVoltage,FilteredCurrent,CoulombCount,Capacity,ConstantK,ConstantA,ConstantB);

end
